simulink model "sedemo_batch_production"  (Simulink 7.5)
settings: Solver=VariableStepDiscrete  StartTime=0.0  StopTime=1000  MaxStep=inf  RelTol=1e-3
PreLoadFcn:
  | assignin('base','AGenerationPeriod',10);
  | assignin('base','AServiceTimeWater',10);
  | assignin('base','AServiceTimeHeat',20);
  | assignin('base','AServiceTimeColor',3);
  | assignin('base','AServiceTimeParticle',5);
  | assignin('base','AServiceTimeStir',10);
  | assignin('base','AServiceTimeDrain',10);
  | assignin('base','BGenerationPeriod',15);
  | assignin('base','BServiceTimeWater',15);
  | assignin('base','BServiceTimeHeat',30);
  | assignin('base','BServiceTimeColor',6);
  | assignin('base','BServiceTimeParticle',10);
  | assignin('base','BServiceTimeStir',20);
  | assignin('base','BServiceTimeDrain',15);
  | assignin('base','NumberOfBatchReactors',10);
  | assignin('base','NumberOfWater',2);
  | assignin('base','NumberOfHeat',3);
  | assignin('base','NumberOfDrain',1);
undefined symbols (not defined in the file or in its folder): AGenerationPeriod, BGenerationPeriod, des_subsystemblock, des_subsysteminport, des_subsystemoutport, des_subsystemsupportblock, NumberOfBatchReactors
libraries: simeventssink1 x12, simeventsserver1 x6, simeventsqueue1 x5, simeventstranslate1 x4, simeventsgenerators1 x3, simeventsrouting1 x3, simeventsentitymanage1 x2, simeventsattributes2 x2, simulink x1, simeventsinfo x1
CloseFcn:
  | clear AGenerationPeriod AServiceTimeWater AServiceTimeHeat AServiceTimeColor AServiceTimeParticle AServiceTimeStir AServiceTimeDrain BGenerationPeriod BServiceTimeWater BServiceTimeHeat BServiceTimeColor BServiceTimeParticle BServiceTimeStir BServiceTimeDrain NumberOfBatchReactors NumberOfHeat NumberOfWater NumberOfDrain;
settings Model: Creator=The MathWorks Inc.
settings DataIOCC: SaveOutput=off  SaveTime=off
settings OptimizationCC: EfficientMapNaN2IntZero=off
settings DebuggingCC: AlgebraicLoopMsg=error  SolverPrmCheckMsg=none  StrictBusMsg=Warning
settings SimEventsCC: propDiagAttribOutput=1  propDiagFcnCallOutput=1  propDiagStatOutput=0

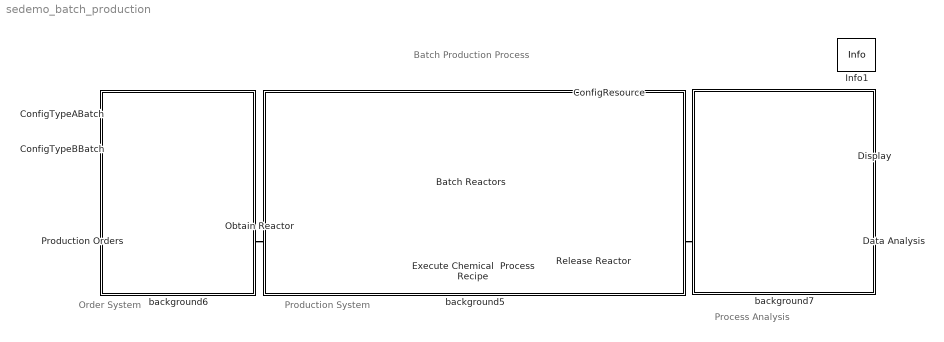
== system sedemo_batch_production ==
  note: Batch Production Process
  note: Production System
  note: Order System
  note: Process Analysis
  Batch Reactors : Subsystem
  ConfigResource : Subsystem  mask{NumBatchReactor=10, NumWater=2, NumHeat=3, NumDrain=1}
      mask prompts: NumBatchReactor "Number of batch reactors:"; NumWater "Capacity of water supply (number of reactors that can access simultaneously):"; NumHeat "Capacity of heat supply (number of reactors that can access simultaneously):"; NumDrain "Capacity of draining facility (number of reactors that can access simultaneously):"
      mask init:
      | assignin('base','NumberOfBatchReactors',NumBatchReactor);
      | assignin('base','NumberOfWater',NumWater);
      | assignin('base','NumberOfHeat',NumHeat);
      | assignin('base','NumberOfDrain',NumDrain);
      mask Display: disp('Double click here to configure\nresource capacity')
  ConfigTypeABatch : Subsystem  mask(Type A batch){AGenPeriod=10, ADelayWater=10, ADelayHeat=20, ADelayColor=3, ADelayParticle=5, ADelayStir=10, ADelayDrain=10}
      mask prompts: AGenPeriod "Order generation period of type A batch:"; ADelayWater "Time needed to add water:"; ADelayHeat "Time needed to heat up:"; ADelayColor "Time needed to add color:"; ADelayParticle "Time needed to add particles:"; ADelayStir "Time needed for agitation:"; ADelayDrain "Time needed to drain:"
      mask init:
      | assignin('base','AGenerationPeriod',AGenPeriod);
      | assignin('base','AServiceTimeWater',ADelayWater);
      | assignin('base','AServiceTimeHeat',ADelayHeat);
      | assignin('base','AServiceTimeColor',ADelayColor);
      | assignin('base','AServiceTimeParticle',ADelayParticle);
      | assignin('base','AServiceTimeStir',ADelayStir);
      | assignin('base','AServiceTimeDrain',ADelayDrain);
      mask Display: disp('Double click here to configure\ntype A batch')
  ConfigTypeBBatch : Subsystem  mask(Type B Batch){BGenPeriod=15, BDelayWater=15, BDelayHeat=30, BDelayColor=6, BDelayParticle=10, BDelayStir=20, BDelayDrain=15}
      mask prompts: BGenPeriod "Order generation period of type B batch:"; BDelayWater "Time needed to add water:"; BDelayHeat "Time needed to heat up:"; BDelayColor "Time needed to add color:"; BDelayParticle "Time needed to add particles:"; BDelayStir "Time needed for agitation:"; BDelayDrain "Time needed to drain:"
      mask init:
      | assignin('base','BGenerationPeriod',BGenPeriod);
      | assignin('base','BServiceTimeWater',BDelayWater);
      | assignin('base','BServiceTimeHeat',BDelayHeat);
      | assignin('base','BServiceTimeColor',BDelayColor);
      | assignin('base','BServiceTimeParticle',BDelayParticle);
      | assignin('base','BServiceTimeStir',BDelayStir);
      | assignin('base','BServiceTimeDrain',BDelayDrain);
      mask Display: disp('Double click here to configure\ntype B batch')
  Data Analysis : Subsystem
  Display : Display
  Execute Chemical  Process Recipe : Subsystem
      mask Display: image(imread('sedemo_batch_reactor.jpg'));
  Info1 : simeventsinfo/Info  SystemSampleTime=-1
  Obtain Reactor : simeventsentitymanage1/Entity Combiner  Priority=1  SystemSampleTime=-1  NumberInputPorts=2  RetainComponentEntities=on  AttributeAccessibility=on  TimerAccessibility=on  AttributeCopied=on  TimerCopied=on  StatNumberDeparted=Off  EvaluatedNumPorts=2
  Production Orders : Subsystem
  Release Reactor : simeventsentitymanage1/Entity Splitter  Priority=1  SystemSampleTime=-1  NumberOutputPorts=2  SplitEntityWhen=All entity output ports are not blocked  OutputPortPrecedence=OUT1 port  InitialSeed=56789  ActionUponPortMismatch=Continue  ActionUponBlocking=Discard entity  StatNumberArrived=Off  StatNumberDeparted=Off  EvaluatedNumPorts=2
  background5 : Subsystem
      mask Display: disp('')
  background6 : Subsystem
      mask Display: disp('')
  background7 : Subsystem
      mask Display:
      | text(18,170,'Reactor util:');
      | text(18,150,'Water util:');
      | text(18,130,'Heat util:');
      | text(18,110,'Drain util:');
  wires:
  Data Analysis/1(ResourceUtil) -> Display/1
  connections:
  Obtain Reactor/RConn1 -- Execute Chemical  Process Recipe/LConn1
  Execute Chemical  Process Recipe/RConn1 -- Release Reactor/LConn1
  Obtain Reactor/LConn1 -- Batch Reactors/RConn1
  Batch Reactors/LConn1 -- Release Reactor/RConn1
  Release Reactor/RConn2 -- Data Analysis/LConn1
  Production Orders/RConn1 -- Obtain Reactor/LConn2

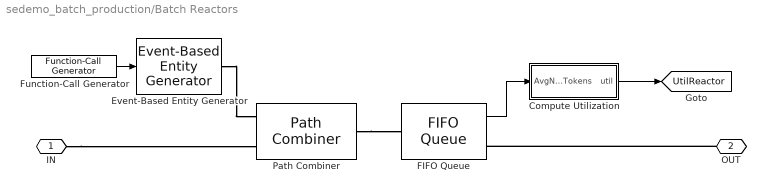
== system sedemo_batch_production/Batch Reactors ==
  Compute Utilization : Subsystem
  Event-Based Entity Generator : simeventsgenerators1/Entity Generators/Event-Based Entity Generator  Priority=1  DialogController=des_ddg_create  DialogControllerArgs=DataTag10  SystemSampleTime=-1  GenerateEntitiesUpon=Function call from port fcn  SignalEdgeType=Rising  SpecifyEventPriority=off  PriorityEntityGeneration=300  GenerateEntityAtSimulationStart=on  AllowBlocking=on  ResponseDuringBlockage=Discard generated entities  EntityType=Blank  StatNumberDeparted=Off  StatPendingEntity=Off  StatAverageIntergenerationTime=Off
  FIFO Queue : simeventsqueue1/FIFO Queue  Priority=1  SystemSampleTime=-1  Capacity=Inf  EnableTOPort=off  StatNumberDeparted=Off  StatNumberInBlock=Off  StatPendingEntity=Off  StatAverageWait=Off  StatAverageQueueLength=On  StatNumberTimedout=Off
  Function-Call Generator : simulink/Ports & Subsystems/Function-Call Generator  sample_time=1e8  numberOfIterations=NumberOfBatchReactors
  Path Combiner : simeventsrouting1/Path Combiner  Priority=1  SystemSampleTime=-1  NumberInputPorts=2  InputPortPrecedence=IN1 port  InitialSeed=45675  SpecifyEventPriority=off  PriorityPathCombinerPortPrecedenceSelection=4100  StatNumberDeparted=Off  StatLastArrivalPort=Off  EvaluatedNumPorts=2
  IN : PMIOPort  Port=1  Side=Left
  OUT : PMIOPort  Port=2  Side=Right
  tag scope: UtilReactor=global
  wires:
  Function-Call Generator/1 -> Event-Based Entity Generator/1
  FIFO Queue/1 -> Compute Utilization/1(AvgNumTokens)
  Compute Utilization/1(util) -> [UtilReactor]
  connections:
  OUT/RConn1 -- FIFO Queue/RConn1
  Path Combiner/RConn1 -- FIFO Queue/LConn1
  Event-Based Entity Generator/RConn1 -- Path Combiner/LConn1
  IN/RConn1 -- Path Combiner/LConn2

== system sedemo_batch_production/ConfigResource ==

== system sedemo_batch_production/ConfigTypeABatch ==

== system sedemo_batch_production/ConfigTypeBBatch ==

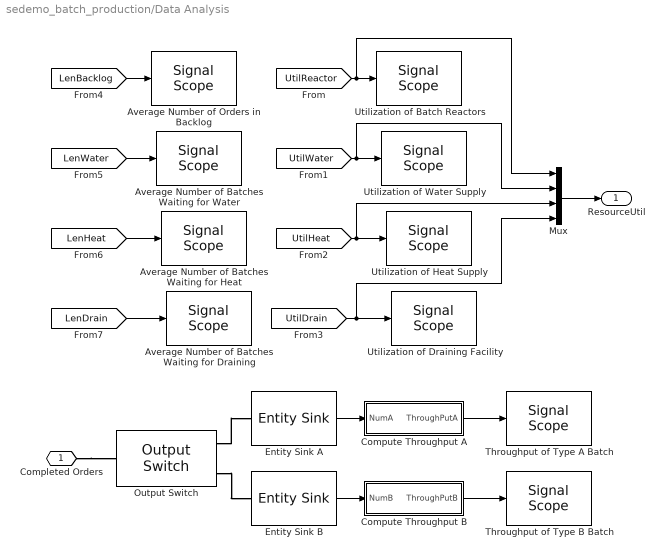
== system sedemo_batch_production/Data Analysis ==
  Average Number of Batches Waiting for Draining : simeventssink1/Signal Scope  Priority=1  SystemSampleTime=-1  PlotType=Stair  InputType=Signal  NumInputs=1  AttributeNameY=Count  XInputOptionSignal=Event time  XInputOptionEntity=Event time  AttributeNameX=Count  EnableEntityOutport=on  XMin=0  XMax=1000  XLimitExceededOption=Stretch axis limits  YLimitExceededOption=Stretch axis limits  AxisGrid=on  AxisLegend=off  LineDisables=""  LineColors=b  LineStyles=-  LineMarkers=None  OpenScopeAtSimStart=on  Title=Avg Num of Batches Waiting for Draining  YLabel=Count  XLabel=Time  FigurePosition=[50 32 259 136]  AxisZoom=off  DataStoreOption=Limited  DataPointsLimit=10000  StatNumberArrived=Off  ShowCountPlotted=off  ShowToolbar=off
      settings: YMin=0  YMax=2
  Average Number of Batches Waiting for Heat : simeventssink1/Signal Scope  Priority=1  SystemSampleTime=-1  PlotType=Stair  InputType=Signal  NumInputs=1  AttributeNameY=Count  XInputOptionSignal=Event time  XInputOptionEntity=Event time  AttributeNameX=Count  EnableEntityOutport=on  XMin=0  XMax=1000  XLimitExceededOption=Stretch axis limits  YLimitExceededOption=Stretch axis limits  AxisGrid=on  AxisLegend=off  LineDisables=""  LineColors="0  1  0"  LineStyles=-  LineMarkers=None  OpenScopeAtSimStart=on  Title=Avg Num of Batches waiting for Heat  YLabel=Count  XLabel=Time  FigurePosition=[50 216 259 136]  AxisZoom=off  DataStoreOption=Limited  DataPointsLimit=10000  StatNumberArrived=Off  ShowCountPlotted=off  ShowToolbar=off
      settings: YMin=0  YMax=2
  Average Number of Batches Waiting for Water : simeventssink1/Signal Scope  Priority=1  SystemSampleTime=-1  PlotType=Stair  InputType=Signal  NumInputs=1  AttributeNameY=Count  XInputOptionSignal=Event time  XInputOptionEntity=Event time  AttributeNameX=Count  EnableEntityOutport=on  XMin=0  XMax=1000  XLimitExceededOption=Stretch axis limits  YLimitExceededOption=Stretch axis limits  AxisGrid=on  AxisLegend=off  LineDisables=""  LineColors="1  0  1"  LineStyles=-  LineMarkers=None  OpenScopeAtSimStart=on  Title=Avg Num of Batches Waiting for Water  YLabel=Count  XLabel=Time  FigurePosition=[52 399 258 136]  AxisZoom=off  DataStoreOption=Limited  DataPointsLimit=10000  StatNumberArrived=Off  ShowCountPlotted=off  ShowToolbar=off
      settings: YMin=0  YMax=2
  Average Number of Orders in Backlog : simeventssink1/Signal Scope  Priority=1  SystemSampleTime=-1  PlotType=Stair  InputType=Signal  NumInputs=1  AttributeNameY=Count  XInputOptionSignal=Event time  XInputOptionEntity=Event time  AttributeNameX=Count  EnableEntityOutport=on  XMin=0  XMax=1000  XLimitExceededOption=Stretch axis limits  YLimitExceededOption=Stretch axis limits  AxisGrid=on  AxisLegend=off  LineDisables=""  LineColors="1  0  0"  LineStyles=-  LineMarkers=None  OpenScopeAtSimStart=on  Title=Average Volume of Order Backlog  YLabel=Count  XLabel=Time  FigurePosition=[51 583 259 136]  AxisZoom=off  DataStoreOption=Limited  DataPointsLimit=10000  StatNumberArrived=Off  ShowCountPlotted=off  ShowToolbar=off
      settings: YMin=0  YMax=2
  Compute Throughput A : Subsystem  LoadFcn=des_subsystemblock(gcb, 'load');  InitFcn=des_subsystemblock(gcb, 'init');  StartFcn=des_subsystemblock(gcb, 'start');  StopFcn=des_subsystemblock(gcb, 'stop');
      settings: CopyFcn=des_subsystemblock(gcb, 'copy');  DeleteFcn=des_subsystemblock(gcb, 'delete');  UndoDeleteFcn=des_subsystemblock(gcb, 'undodelete');  ModelCloseFcn=des_subsystemblock(gcb, 'modelclose');  PreSaveFcn=des_subsystemblock(gcb, 'presave');  NameChangeFcn=des_subsystemblock(gcb, 'namechange');  OpenFcn=des_subsystemblock(gcb, 'open');  ParentCloseFcn=des_subsystemblock(gcb, 'parentclose');  ErrorFcn=des_subsystemerror
      mask Type: Discrete Event Subsystem
      mask Help: helpview(simeventsbhelp);
  Compute Throughput B : Subsystem  LoadFcn=des_subsystemblock(gcb, 'load');  InitFcn=des_subsystemblock(gcb, 'init');  StartFcn=des_subsystemblock(gcb, 'start');  StopFcn=des_subsystemblock(gcb, 'stop');
      settings: CopyFcn=des_subsystemblock(gcb, 'copy');  DeleteFcn=des_subsystemblock(gcb, 'delete');  UndoDeleteFcn=des_subsystemblock(gcb, 'undodelete');  ModelCloseFcn=des_subsystemblock(gcb, 'modelclose');  PreSaveFcn=des_subsystemblock(gcb, 'presave');  NameChangeFcn=des_subsystemblock(gcb, 'namechange');  OpenFcn=des_subsystemblock(gcb, 'open');  ParentCloseFcn=des_subsystemblock(gcb, 'parentclose');  ErrorFcn=des_subsystemerror
      mask Type: Discrete Event Subsystem
      mask Help: helpview(simeventsbhelp);
  Entity Sink A : simeventssink1/Entity Sink  Priority=1  SystemSampleTime=-1  AvailableForArrivals=on  StatNumberArrived=On
  Entity Sink B : simeventssink1/Entity Sink  Priority=1  SystemSampleTime=-1  AvailableForArrivals=on  StatNumberArrived=On
  Mux : Mux
  Output Switch : simeventsrouting1/Output Switch  Priority=1  SystemSampleTime=-1  NumberOutputPorts=2  SwitchingCriterion=From attribute  InitialSeed=34567  AttributeName=TypeOfBatch  InitialConditionsOpt=off  InitialConditions=1  EntityBufferOpt=off  SpecifyEventPriority=off  PriorityOutputSwitchSelectPort=4100  TimeoutPortOpt=off  StatNumberDeparted=Off  StatNumberTimedOut=Off  StatPendingEntity=Off  StatLastDeparturePort=Off  EvaluatedNumPorts=2
  Throughput of Type A Batch : simeventssink1/Signal Scope  Priority=1  SystemSampleTime=-1  PlotType=Stair  InputType=Signal  NumInputs=1  AttributeNameY=Count  XInputOptionSignal=Event time  XInputOptionEntity=Event time  AttributeNameX=Count  EnableEntityOutport=on  XMin=0  XMax=1000  XLimitExceededOption=Stretch axis limits  YLimitExceededOption=Stretch axis limits  AxisGrid=on  AxisLegend=off  LineDisables=""  LineColors=b  LineStyles=-  LineMarkers=None  OpenScopeAtSimStart=on  Title=Throughput of Type A Batch  YLabel=Throughput (batch/sec)  XLabel=Time  FigurePosition=[606 404 285 146]  AxisZoom=off  DataStoreOption=Limited  DataPointsLimit=10000  StatNumberArrived=Off  ShowCountPlotted=off  ShowToolbar=off
      settings: YMin=0  YMax=0.1
  Throughput of Type B Batch : simeventssink1/Signal Scope  Priority=1  SystemSampleTime=-1  PlotType=Stair  InputType=Signal  NumInputs=1  AttributeNameY=Count  XInputOptionSignal=Event time  XInputOptionEntity=Event time  AttributeNameX=Count  EnableEntityOutport=on  XMin=0  XMax=1000  XLimitExceededOption=Stretch axis limits  YLimitExceededOption=Stretch axis limits  AxisGrid=on  AxisLegend=off  LineDisables=""  LineColors=b  LineStyles=-  LineMarkers=None  OpenScopeAtSimStart=on  Title=Throughput of Type B Batch  YLabel=Throughput (batch/sec)  XLabel=Time  FigurePosition=[606 211 285 146]  AxisZoom=off  DataStoreOption=Limited  DataPointsLimit=10000  StatNumberArrived=Off  ShowCountPlotted=off  ShowToolbar=off
      settings: YMin=0  YMax=0.1
  Utilization of Batch Reactors : simeventssink1/Signal Scope  Priority=1  SystemSampleTime=-1  PlotType=Stair  InputType=Signal  NumInputs=1  AttributeNameY=Count  XInputOptionSignal=Event time  XInputOptionEntity=Event time  AttributeNameX=Count  EnableEntityOutport=on  XMin=0  XMax=1000  XLimitExceededOption=Stretch axis limits  YLimitExceededOption=Stretch axis limits  AxisGrid=on  AxisLegend=off  LineDisables=""  LineColors="1  0  0"  LineStyles=-  LineMarkers=None  OpenScopeAtSimStart=on  Title=Utilization of Batch Reactors  YLabel=Utilization  XLabel=Time  FigurePosition=[318 584 264 135]  AxisZoom=off  DataStoreOption=Limited  DataPointsLimit=10000  StatNumberArrived=Off  ShowCountPlotted=off  ShowToolbar=off
      settings: YMin=0  YMax=1.2
  Utilization of Draining Facility : simeventssink1/Signal Scope  Priority=1  SystemSampleTime=-1  PlotType=Stair  InputType=Signal  NumInputs=1  AttributeNameY=Count  XInputOptionSignal=Event time  XInputOptionEntity=Event time  AttributeNameX=Count  EnableEntityOutport=on  XMin=0  XMax=1000  XLimitExceededOption=Stretch axis limits  YLimitExceededOption=Stretch axis limits  AxisGrid=on  AxisLegend=off  LineDisables=""  LineColors=b  LineStyles=-  LineMarkers=None  OpenScopeAtSimStart=on  Title=Utilization of Draining Facility  YLabel=Utilization  XLabel=Time  FigurePosition=[317 33 265 135]  AxisZoom=off  DataStoreOption=Limited  DataPointsLimit=10000  StatNumberArrived=Off  ShowCountPlotted=off  ShowToolbar=off
      settings: YMin=0  YMax=1.2
  Utilization of Heat Supply : simeventssink1/Signal Scope  Priority=1  SystemSampleTime=-1  PlotType=Stair  InputType=Signal  NumInputs=1  AttributeNameY=Count  XInputOptionSignal=Event time  XInputOptionEntity=Event time  AttributeNameX=Count  EnableEntityOutport=on  XMin=0  XMax=1000  XLimitExceededOption=Stretch axis limits  YLimitExceededOption=Stretch axis limits  AxisGrid=on  AxisLegend=off  LineDisables=""  LineColors="0  1  0"  LineStyles=-  LineMarkers=None  OpenScopeAtSimStart=on  Title=Utilization of Heat  YLabel=Utilization  XLabel=Time  FigurePosition=[317 216 265 137]  AxisZoom=off  DataStoreOption=Limited  DataPointsLimit=10000  StatNumberArrived=Off  ShowCountPlotted=off  ShowToolbar=off
      settings: YMin=0  YMax=1.2
  Utilization of Water Supply : simeventssink1/Signal Scope  Priority=1  SystemSampleTime=-1  PlotType=Stair  InputType=Signal  NumInputs=1  AttributeNameY=Count  XInputOptionSignal=Event time  XInputOptionEntity=Event time  AttributeNameX=Count  EnableEntityOutport=on  XMin=0  XMax=1000  XLimitExceededOption=Stretch axis limits  YLimitExceededOption=Stretch axis limits  AxisGrid=on  AxisLegend=off  LineDisables=""  LineColors="1  0  1"  LineStyles=-  LineMarkers=None  OpenScopeAtSimStart=on  Title=Utilization of Water  YLabel=Utilization  XLabel=Time  FigurePosition=[318 401 264 135]  AxisZoom=off  DataStoreOption=Limited  DataPointsLimit=10000  StatNumberArrived=Off  ShowCountPlotted=off  ShowToolbar=off
      settings: YMin=0  YMax=1.2
  Completed Orders : PMIOPort  Port=1  Side=Left
  ResourceUtil : Outport  OutDataType=sfix(16)  OutScaling=2^0
  wires:
  [UtilReactor] -> Utilization of Batch Reactors/1, Mux/1
  [UtilWater] -> Utilization of Water Supply/1, Mux/2
  [UtilDrain] -> Utilization of Draining Facility/1, Mux/4
  [UtilHeat] -> Utilization of Heat Supply/1, Mux/3
  [LenBacklog] -> Average Number of Orders in Backlog/1
  [LenWater] -> Average Number of Batches Waiting for Water/1
  [LenDrain] -> Average Number of Batches Waiting for Draining/1
  [LenHeat] -> Average Number of Batches Waiting for Heat/1
  Entity Sink A/1 -> Compute Throughput A/1(NumA)
  Entity Sink B/1 -> Compute Throughput B/1(NumB)
  Compute Throughput A/1(ThroughPutA) -> Throughput of Type A Batch/1
  Compute Throughput B/1(ThroughPutB) -> Throughput of Type B Batch/1
  Mux/1 -> ResourceUtil/1
  connections:
  Completed Orders/RConn1 -- Output Switch/LConn1
  Output Switch/RConn1 -- Entity Sink A/LConn1
  Output Switch/RConn2 -- Entity Sink B/LConn1

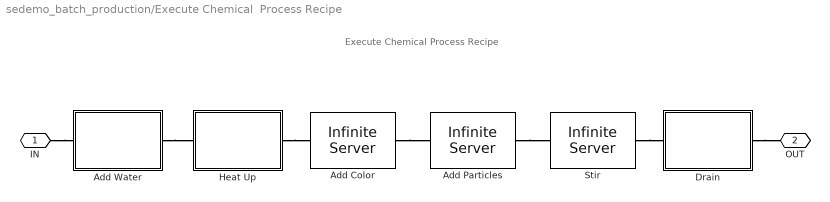
== system sedemo_batch_production/Execute Chemical  Process Recipe ==
  note: Execute Chemical Process Recipe
  Add Color : simeventsserver1/Infinite Server  Priority=1  SystemSampleTime=-1  ServiceTimeFrom=Attribute  ServiceTime=1  AttributeName=ServiceTimeColor  PriorityServiceCompletion=500  EnableTOPort=off  StatNumberDeparted=Off  StatNumberInBlock=Off  StatPendingEntity=Off  StatNumberPending=Off  StatAverageWait=Off  StatNumberTimedout=Off
  Add Particles : simeventsserver1/Infinite Server  Priority=1  SystemSampleTime=-1  ServiceTimeFrom=Attribute  ServiceTime=1  AttributeName=ServiceTimeParticle  PriorityServiceCompletion=500  EnableTOPort=off  StatNumberDeparted=Off  StatNumberInBlock=Off  StatPendingEntity=Off  StatNumberPending=Off  StatAverageWait=Off  StatNumberTimedout=Off
  Add Water : Subsystem
  Drain : Subsystem
  Heat Up : Subsystem
  Stir : simeventsserver1/Infinite Server  Priority=1  SystemSampleTime=-1  ServiceTimeFrom=Attribute  ServiceTime=1  AttributeName=ServiceTimeStir  PriorityServiceCompletion=500  EnableTOPort=off  StatNumberDeparted=Off  StatNumberInBlock=Off  StatPendingEntity=Off  StatNumberPending=Off  StatAverageWait=Off  StatNumberTimedout=Off
  IN : PMIOPort  Port=1  Side=Left
  OUT : PMIOPort  Port=2  Side=Right
  connections:
  Add Color/RConn1 -- Add Particles/LConn1
  Add Particles/RConn1 -- Stir/LConn1
  IN/RConn1 -- Add Water/LConn1
  Add Water/RConn1 -- Heat Up/LConn1
  Heat Up/RConn1 -- Add Color/LConn1
  Stir/RConn1 -- Drain/LConn1
  Drain/RConn1 -- OUT/RConn1

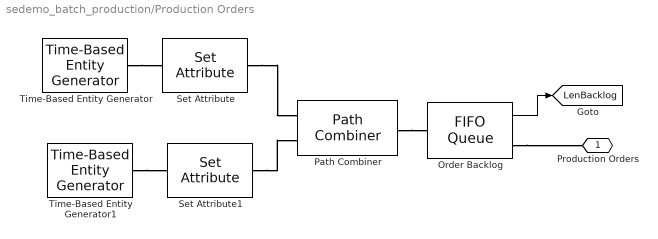
== system sedemo_batch_production/Production Orders ==
  Order Backlog : simeventsqueue1/FIFO Queue  Priority=1  SystemSampleTime=-1  Capacity=Inf  EnableTOPort=off  StatNumberDeparted=Off  StatNumberInBlock=Off  StatPendingEntity=Off  StatAverageWait=Off  StatAverageQueueLength=On  StatNumberTimedout=Off
  Path Combiner : simeventsrouting1/Path Combiner  Priority=1  SystemSampleTime=-1  NumberInputPorts=2  InputPortPrecedence=IN1 port  InitialSeed=45675  SpecifyEventPriority=off  PriorityPathCombinerPortPrecedenceSelection=4100  StatNumberDeparted=Off  StatLastArrivalPort=Off  EvaluatedNumPorts=2
  Set Attribute : simeventsattributes2/Set Attribute  Priority=1  DialogController=des_ddg_create  DialogControllerArgs=DataTag53  SystemSampleTime=-1  AttributeFrom=Dialog|Dialog|Dialog|Dialog|Dialog|Dialog|Dialog  AttributeName=ServiceTimeWater|ServiceTimeHeat|ServiceTimeColor|ServiceTimeParticle|ServiceTimeStir|ServiceTimeDrain|TypeOfBatch  AttributeTreatAsVector=1|1|1|1|1|1|1  AttributeValue=AServiceTimeWater|AServiceTimeHeat|AServiceTimeColor|AServiceTimeParticle|AServiceTimeStir|AServiceTimeDrain|1  AttributeCreate=on  StatNumberDeparted=Off  EvaluatedAttributeValue={AServiceTimeWater;AServiceTimeHeat;AServiceTimeColor;AServiceTimeParticle;AServiceTimeStir;AServiceTimeDrain;1}
  Set Attribute1 : simeventsattributes2/Set Attribute  Priority=1  DialogController=des_ddg_create  DialogControllerArgs=DataTag55  SystemSampleTime=-1  AttributeFrom=Dialog|Dialog|Dialog|Dialog|Dialog|Dialog|Dialog  AttributeName=ServiceTimeWater|ServiceTimeHeat|ServiceTimeColor|ServiceTimeParticle|ServiceTimeStir|ServiceTimeDrain|TypeOfBatch  AttributeTreatAsVector=1|1|1|1|1|1|1  AttributeValue=BServiceTimeWater|BServiceTimeHeat|BServiceTimeColor|BServiceTimeParticle|BServiceTimeStir|BServiceTimeDrain|2  AttributeCreate=on  StatNumberDeparted=Off  EvaluatedAttributeValue={BServiceTimeWater;BServiceTimeHeat;BServiceTimeColor;BServiceTimeParticle;BServiceTimeStir;BServiceTimeDrain;2}
  Time-Based Entity Generator : simeventsgenerators1/Entity Generators/Time-Based Entity Generator  Priority=1  DialogController=des_ddg_create  DialogControllerArgs=DataTag57  SystemSampleTime=-1  GenerateEntitiesUpon=Intergeneration time from dialog  Distribution=Constant  Minimum=0  Maximum=1  Mean=1  InitialSeed=12345  Period=AGenerationPeriod  PriorityEntityGeneration=300  GenerateEntityAtSimulationStart=off  ResponseWhenBlocked=Pause generation  ResponseWhenUnblocked=Immediate restart  EntityType=Blank  StatNumberDeparted=Off  StatPendingEntity=Off  StatAverageIntergenerationTime=Off
  Time-Based Entity Generator1 : simeventsgenerators1/Entity Generators/Time-Based Entity Generator  Priority=1  DialogController=des_ddg_create  DialogControllerArgs=DataTag59  SystemSampleTime=-1  GenerateEntitiesUpon=Intergeneration time from dialog  Distribution=Constant  Minimum=0  Maximum=1  Mean=1  InitialSeed=12345  Period=BGenerationPeriod  PriorityEntityGeneration=300  GenerateEntityAtSimulationStart=off  ResponseWhenBlocked=Pause generation  ResponseWhenUnblocked=Immediate restart  EntityType=Blank  StatNumberDeparted=Off  StatPendingEntity=Off  StatAverageIntergenerationTime=Off
  Production Orders : PMIOPort  Port=1  Side=Right
  tag scope: LenBacklog=global
  wires:
  Order Backlog/1 -> [LenBacklog]
  connections:
  Set Attribute/RConn1 -- Path Combiner/LConn1
  Set Attribute1/RConn1 -- Path Combiner/LConn2
  Time-Based Entity Generator/RConn1 -- Set Attribute/LConn1
  Time-Based Entity Generator1/RConn1 -- Set Attribute1/LConn1
  Path Combiner/RConn1 -- Order Backlog/LConn1
  Order Backlog/RConn1 -- Production Orders/RConn1

== system sedemo_batch_production/background5 ==

== system sedemo_batch_production/background6 ==

== system sedemo_batch_production/background7 ==

== system sedemo_batch_production/Batch Reactors/Compute Utilization ==
  AvgNumTokens : Inport
  Constant : Constant  Value=NumberOfBatchReactors  OutDataType=sfix(16)  OutScaling=2^0
  Discrete Event Subsystem : Subsystem  LoadFcn=des_subsystemblock(gcb, 'load');  InitFcn=des_subsystemblock(gcb, 'init');  StartFcn=des_subsystemblock(gcb, 'start');  StopFcn=des_subsystemblock(gcb, 'stop');
      settings: CopyFcn=des_subsystemblock(gcb, 'copy');  DeleteFcn=des_subsystemblock(gcb, 'delete');  UndoDeleteFcn=des_subsystemblock(gcb, 'undodelete');  ModelCloseFcn=des_subsystemblock(gcb, 'modelclose');  PreSaveFcn=des_subsystemblock(gcb, 'presave');  NameChangeFcn=des_subsystemblock(gcb, 'namechange');  OpenFcn=des_subsystemblock(gcb, 'open');  ParentCloseFcn=des_subsystemblock(gcb, 'parentclose');  ErrorFcn=des_subsystemerror
      mask Type: Discrete Event Subsystem
      mask Help: helpview(simeventsbhelp);
  util : Outport
  wires:
  Constant/1 -> Discrete Event Subsystem/1(Capacity)
  Discrete Event Subsystem/1(util) -> util/1
  AvgNumTokens/1 -> Discrete Event Subsystem/2(AvgNumTokens)

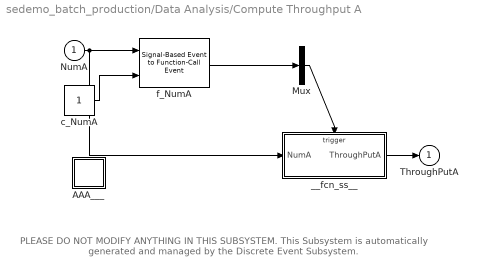
== system sedemo_batch_production/Data Analysis/Compute Throughput A ==
  note: PLEASE DO NOT MODIFY ANYTHING IN THIS SUBSYSTEM.
      | This Subsystem is automatically generated and
      | managed by the Discrete Event Subsystem.
  NumA : Inport  DataType=double  OutDataType=sfix(16)  OutScaling=2^0  OutDataTypeStr=double
  AAA___ : Subsystem  LoadFcn=des_subsystemsupportblock(gcb, 'load');  InitFcn=des_subsystemsupportblock(gcb, 'init');  StartFcn=des_subsystemsupportblock(gcb, 'start');  StopFcn=des_subsystemsupportblock(gcb, 'stop');
      settings: CopyFcn=des_subsystemsupportblock(gcb, 'copy');  DeleteFcn=des_subsystemsupportblock(gcb, 'delete');  UndoDeleteFcn=des_subsystemsupportblock(gcb, 'undodelete');  ModelCloseFcn=des_subsystemsupportblock(gcb, 'modelclose');  PreSaveFcn=des_subsystemsupportblock(gcb, 'presave');  NameChangeFcn=des_subsystemsupportblock(gcb, 'namechange');  OpenFcn=des_subsystemsupportblock(gcb, 'open');  ParentCloseFcn=des_subsystemsupportblock(gcb, 'parentclose');
  Mux : Mux  Inputs=1
  __fcn_ss__ : Subsystem  TreatAsAtomicUnit=on
      settings: PropExecContextOutsideSubsystem=on
  c_NumA : Constant  OutDataType=sfix(16)  OutScaling=2^0
  f_NumA : simeventstranslate1/Signal-Based Event to Function-Call Event  Priority=1  SystemSampleTime=-1  GenerateFunctionCallUpon=Sample time hit from port ts  SignalEdgeOption=Rising  EnableE1Port=on  EnableF2Port=off  EnableE2Port=off  SpecifyEventPriority=off  PriorityFunctionCall=20  FunctionCallDelayFrom=Dialog  DelayFunctionCall=0  StatNumberF1Calls=Off  StatNumberF2Calls=Off  MaskBlockType=DESS_EVENT_PORT
  ThroughPutA : Outport  OutDataType=sfix(16)  OutScaling=2^0
  wires:
  __fcn_ss__/1(ThroughPutA) -> ThroughPutA/1
  f_NumA/1 -> Mux/1
  c_NumA/1 -> f_NumA/2
  Mux/1 -> __fcn_ss__/Trigger
  NumA/1 -> f_NumA/1, __fcn_ss__/1(NumA)

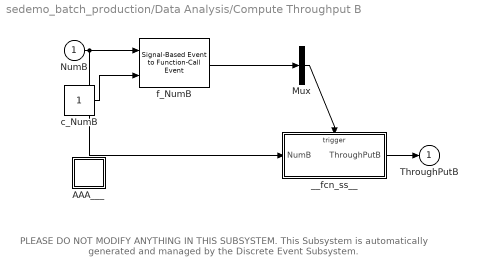
== system sedemo_batch_production/Data Analysis/Compute Throughput B ==
  note: PLEASE DO NOT MODIFY ANYTHING IN THIS SUBSYSTEM.
      | This Subsystem is automatically generated and
      | managed by the Discrete Event Subsystem.
  NumB : Inport  DataType=double  OutDataType=sfix(16)  OutScaling=2^0  OutDataTypeStr=double
  AAA___ : Subsystem  LoadFcn=des_subsystemsupportblock(gcb, 'load');  InitFcn=des_subsystemsupportblock(gcb, 'init');  StartFcn=des_subsystemsupportblock(gcb, 'start');  StopFcn=des_subsystemsupportblock(gcb, 'stop');
      settings: CopyFcn=des_subsystemsupportblock(gcb, 'copy');  DeleteFcn=des_subsystemsupportblock(gcb, 'delete');  UndoDeleteFcn=des_subsystemsupportblock(gcb, 'undodelete');  ModelCloseFcn=des_subsystemsupportblock(gcb, 'modelclose');  PreSaveFcn=des_subsystemsupportblock(gcb, 'presave');  NameChangeFcn=des_subsystemsupportblock(gcb, 'namechange');  OpenFcn=des_subsystemsupportblock(gcb, 'open');  ParentCloseFcn=des_subsystemsupportblock(gcb, 'parentclose');
  Mux : Mux  Inputs=1
  __fcn_ss__ : Subsystem  TreatAsAtomicUnit=on
      settings: PropExecContextOutsideSubsystem=on
  c_NumB : Constant  OutDataType=sfix(16)  OutScaling=2^0
  f_NumB : simeventstranslate1/Signal-Based Event to Function-Call Event  Priority=1  SystemSampleTime=-1  GenerateFunctionCallUpon=Sample time hit from port ts  SignalEdgeOption=Rising  EnableE1Port=on  EnableF2Port=off  EnableE2Port=off  SpecifyEventPriority=off  PriorityFunctionCall=20  FunctionCallDelayFrom=Dialog  DelayFunctionCall=0  StatNumberF1Calls=Off  StatNumberF2Calls=Off  MaskBlockType=DESS_EVENT_PORT
  ThroughPutB : Outport  OutDataType=sfix(16)  OutScaling=2^0
  wires:
  Mux/1 -> __fcn_ss__/Trigger
  c_NumB/1 -> f_NumB/2
  f_NumB/1 -> Mux/1
  __fcn_ss__/1(ThroughPutB) -> ThroughPutB/1
  NumB/1 -> f_NumB/1, __fcn_ss__/1(NumB)

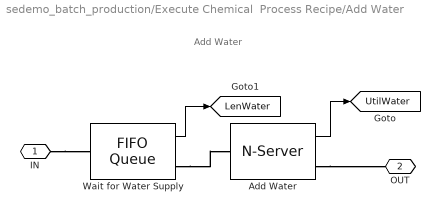
== system sedemo_batch_production/Execute Chemical  Process Recipe/Add Water ==
  note: Add Water
  Add Water : simeventsserver1/N-Server  Priority=1  SystemSampleTime=-1  NumberOfServers=NumberOfWater  ServiceTimeFrom=Attribute  ServiceTime=1  AttributeName=ServiceTimeWater  PriorityServiceCompletion=500  EnableTOPort=off  StatNumberDeparted=Off  StatNumberInBlock=Off  StatPendingEntity=Off  StatNumberPending=Off  StatAverageWait=Off  StatUtilization=On  StatNumberTimedout=Off
  Wait for Water Supply : simeventsqueue1/FIFO Queue  Priority=1  SystemSampleTime=-1  Capacity=Inf  EnableTOPort=off  StatNumberDeparted=Off  StatNumberInBlock=Off  StatPendingEntity=Off  StatAverageWait=Off  StatAverageQueueLength=On  StatNumberTimedout=Off
  IN : PMIOPort  Port=1  Side=Left
  OUT : PMIOPort  Port=2  Side=Right
  tag scope: LenWater=global, UtilWater=global
  wires:
  Add Water/1 -> [UtilWater]
  Wait for Water Supply/1 -> [LenWater]
  connections:
  Add Water/RConn1 -- OUT/RConn1
  IN/RConn1 -- Wait for Water Supply/LConn1
  Wait for Water Supply/RConn1 -- Add Water/LConn1

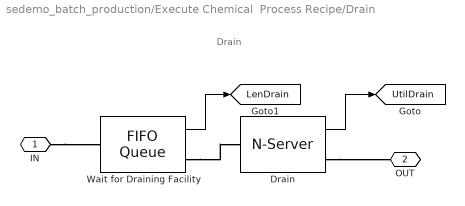
== system sedemo_batch_production/Execute Chemical  Process Recipe/Drain ==
  note: Drain
  Drain : simeventsserver1/N-Server  Priority=1  SystemSampleTime=-1  NumberOfServers=NumberOfDrain  ServiceTimeFrom=Attribute  ServiceTime=1  AttributeName=ServiceTimeDrain  PriorityServiceCompletion=500  EnableTOPort=off  StatNumberDeparted=Off  StatNumberInBlock=Off  StatPendingEntity=Off  StatNumberPending=Off  StatAverageWait=Off  StatUtilization=On  StatNumberTimedout=Off
  Wait for Draining Facility : simeventsqueue1/FIFO Queue  Priority=1  SystemSampleTime=-1  Capacity=Inf  EnableTOPort=off  StatNumberDeparted=Off  StatNumberInBlock=Off  StatPendingEntity=Off  StatAverageWait=Off  StatAverageQueueLength=On  StatNumberTimedout=Off
  IN : PMIOPort  Port=1  Side=Left
  OUT : PMIOPort  Port=2  Side=Right
  tag scope: LenDrain=global, UtilDrain=global
  wires:
  Drain/1 -> [UtilDrain]
  Wait for Draining Facility/1 -> [LenDrain]
  connections:
  IN/RConn1 -- Wait for Draining Facility/LConn1
  Wait for Draining Facility/RConn1 -- Drain/LConn1
  Drain/RConn1 -- OUT/RConn1

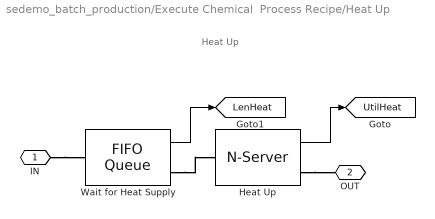
== system sedemo_batch_production/Execute Chemical  Process Recipe/Heat Up ==
  note: Heat Up
  Heat Up : simeventsserver1/N-Server  Priority=1  SystemSampleTime=-1  NumberOfServers=NumberOfHeat  ServiceTimeFrom=Attribute  ServiceTime=1  AttributeName=ServiceTimeHeat  PriorityServiceCompletion=500  EnableTOPort=off  StatNumberDeparted=Off  StatNumberInBlock=Off  StatPendingEntity=Off  StatNumberPending=Off  StatAverageWait=Off  StatUtilization=On  StatNumberTimedout=Off
  Wait for Heat Supply : simeventsqueue1/FIFO Queue  Priority=1  SystemSampleTime=-1  Capacity=Inf  EnableTOPort=off  StatNumberDeparted=Off  StatNumberInBlock=Off  StatPendingEntity=Off  StatAverageWait=Off  StatAverageQueueLength=On  StatNumberTimedout=Off
  IN : PMIOPort  Port=1  Side=Left
  OUT : PMIOPort  Port=2  Side=Right
  tag scope: LenHeat=global, UtilHeat=global
  wires:
  Heat Up/1 -> [UtilHeat]
  Wait for Heat Supply/1 -> [LenHeat]
  connections:
  Heat Up/RConn1 -- OUT/RConn1
  Wait for Heat Supply/RConn1 -- Heat Up/LConn1
  IN/RConn1 -- Wait for Heat Supply/LConn1

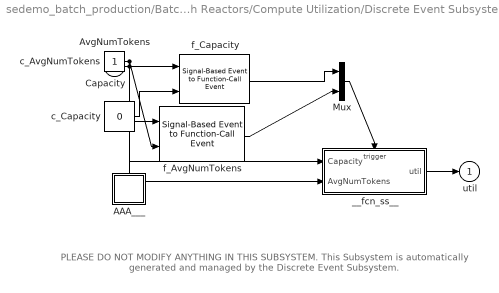
== system sedemo_batch_production/Batch Reactors/Compute Utilization/Discrete Event Subsystem ==
  note: PLEASE DO NOT MODIFY ANYTHING IN THIS SUBSYSTEM.
      | This Subsystem is automatically generated and
      | managed by the Discrete Event Subsystem.
  Capacity : Inport  DataType=double  OutDataType=sfix(16)  OutScaling=2^0  OutDataTypeStr=double
  AvgNumTokens : Inport  Port=2  DataType=double  OutDataTypeStr=double
  AAA___ : Subsystem  LoadFcn=des_subsystemsupportblock(gcb, 'load');  InitFcn=des_subsystemsupportblock(gcb, 'init');  StartFcn=des_subsystemsupportblock(gcb, 'start');  StopFcn=des_subsystemsupportblock(gcb, 'stop');
      settings: CopyFcn=des_subsystemsupportblock(gcb, 'copy');  DeleteFcn=des_subsystemsupportblock(gcb, 'delete');  UndoDeleteFcn=des_subsystemsupportblock(gcb, 'undodelete');  ModelCloseFcn=des_subsystemsupportblock(gcb, 'modelclose');  PreSaveFcn=des_subsystemsupportblock(gcb, 'presave');  NameChangeFcn=des_subsystemsupportblock(gcb, 'namechange');  OpenFcn=des_subsystemsupportblock(gcb, 'open');  ParentCloseFcn=des_subsystemsupportblock(gcb, 'parentclose');
  Mux : Mux  Inputs=2
  __fcn_ss__ : Subsystem  TreatAsAtomicUnit=on
      settings: PropExecContextOutsideSubsystem=on
  c_AvgNumTokens : Constant
  c_Capacity : Constant  Value=0  OutDataType=sfix(16)  OutScaling=2^0
  f_AvgNumTokens : simeventstranslate1/Signal-Based Event to Function-Call Event  Priority=1  SystemSampleTime=-1  GenerateFunctionCallUpon=Sample time hit from port ts  SignalEdgeOption=Rising  EnableE1Port=on  EnableF2Port=off  EnableE2Port=off  SpecifyEventPriority=off  PriorityFunctionCall=20  FunctionCallDelayFrom=Dialog  DelayFunctionCall=0  StatNumberF1Calls=Off  StatNumberF2Calls=Off  MaskBlockType=DESS_EVENT_PORT
  f_Capacity : simeventstranslate1/Signal-Based Event to Function-Call Event  Priority=1  SystemSampleTime=-1  GenerateFunctionCallUpon=Sample time hit from port ts  SignalEdgeOption=Rising  EnableE1Port=on  EnableF2Port=off  EnableE2Port=off  SpecifyEventPriority=off  PriorityFunctionCall=20  FunctionCallDelayFrom=Dialog  DelayFunctionCall=0  StatNumberF1Calls=Off  StatNumberF2Calls=Off  MaskBlockType=DESS_DATA_PORT
  util : Outport  OutDataType=sfix(16)  OutScaling=2^0
  wires:
  Capacity/1 -> __fcn_ss__/1(Capacity), f_Capacity/1
  __fcn_ss__/1(util) -> util/1
  f_Capacity/1 -> Mux/1
  c_Capacity/1 -> f_Capacity/2
  Mux/1 -> __fcn_ss__/Trigger
  f_AvgNumTokens/1 -> Mux/2
  c_AvgNumTokens/1 -> f_AvgNumTokens/2
  AvgNumTokens/1 -> f_AvgNumTokens/1, __fcn_ss__/2(AvgNumTokens)

== system sedemo_batch_production/Data Analysis/Compute Throughput A/AAA___ ==

== system sedemo_batch_production/Data Analysis/Compute Throughput A/__fcn_ss__ ==
  NumA : Inport  LoadFcn=des_subsysteminport(gcb, 'load');  InitFcn=des_subsysteminport(gcb, 'init');  StartFcn=des_subsysteminport(gcb, 'start');  StopFcn=des_subsysteminport(gcb, 'stop');  OutDataType=sfix(16)  OutScaling=2^0  mask(Discrete Event Inport){PermitSubsystemEvents=on, TypeOfEvent=Sample time hit, SignalEdgeOption=Rising, SpecifyEventPriority=off, PrioritySubsystemEvent=20}
      mask prompts: PermitSubsystemEvents "Execute subsystem upon signal-based events"; TypeOfEvent "Type of signal-based event:"; SignalEdgeOption "Type of change in signal value:"; SpecifyEventPriority "Resolve simultaneous signal updates according to event priority"; PrioritySubsystemEvent "Event priority:"
      mask help: Input port for a Discrete Event Subsystem block. This block can conditionally execute the subsystem upon signal-based events that meet specified criteria.
      mask init:
      | des_subsystemmask(gcb, 'init','apply')
      settings: CopyFcn=des_subsysteminport(gcb, 'copy');  DeleteFcn=des_subsysteminport(gcb, 'delete');  UndoDeleteFcn=des_subsysteminport(gcb, 'undodelete');  ModelCloseFcn=des_subsysteminport(gcb, 'modelclose');  PreSaveFcn=des_subsysteminport(gcb, 'presave');  NameChangeFcn=des_subsysteminport(gcb, 'namechange');  ParentCloseFcn=des_subsysteminport(gcb, 'parentclose');
      mask Help: helpview(simeventsbhelp);
      mask StyleString: checkbox,popup(Change in signal|Trigger|Sample time hit),popup(Rising|Falling|Either),checkbox,edit
      mask CallbackString: des_subsystemmask(gcb, 'cbPermitSubsystemEvents', 'noapply');|des_subsystemmask(gcb,'cbTypeOfEvent','noapply');||des_subsystemmask(gcb, 'cbSpecifyEventPriority', 'noapply');|
  Subsystem Configuration : TriggerPort  TriggerType=function-call
      settings: CopyFcn=des_subsystemconfigblock(gcb, 'copy');  DeleteFcn=des_subsystemconfigblock(gcb, 'delete');  UndoDeleteFcn=des_subsystemconfigblock(gcb, 'undodelete');
      mask Type: Subsystem Configuration
      mask Description: Configuration for a Discrete Event Subsystem block. Every discrete event subsystem window must contain exactly one copy of this configuration block. Do not delete this block.
      mask Help: helpview(simeventsbhelp);
      mask Display: disp('Do Not Delete');
  Digital Clock : DigitalClock  SampleTime=-1
  Divide : Product  Inputs=*/  OutDataType=sfix(16)  OutScaling=2^-10
  ThroughPutA : Outport  LoadFcn=des_subsystemoutport(gcb, 'load');  InitFcn=des_subsystemoutport(gcb, 'init');  StartFcn=des_subsystemoutport(gcb, 'start');  StopFcn=des_subsystemoutport(gcb, 'stop');  OutDataType=sfix(16)  OutScaling=2^0
      settings: CopyFcn=des_subsystemoutport(gcb, 'copy');  DeleteFcn=des_subsystemoutport(gcb, 'delete');  UndoDeleteFcn=des_subsystemoutport(gcb, 'undodelete');  ModelCloseFcn=des_subsystemoutport(gcb, 'modelclose');  PreSaveFcn=des_subsystemoutport(gcb, 'presave');  NameChangeFcn=des_subsystemoutport(gcb, 'namechange');  ParentCloseFcn=des_subsystemoutport(gcb, 'parentclose');
      mask Type: Discrete Event Outport
      mask Description: Provide an output port for a Discrete Event Subsystem block.
      mask Help: helpview(simeventsbhelp);
  wires:
  NumA/1 -> Divide/1
  Divide/1 -> ThroughPutA/1
  Digital Clock/1 -> Divide/2

== system sedemo_batch_production/Data Analysis/Compute Throughput B/AAA___ ==

== system sedemo_batch_production/Data Analysis/Compute Throughput B/__fcn_ss__ ==
  NumB : Inport  LoadFcn=des_subsysteminport(gcb, 'load');  InitFcn=des_subsysteminport(gcb, 'init');  StartFcn=des_subsysteminport(gcb, 'start');  StopFcn=des_subsysteminport(gcb, 'stop');  OutDataType=sfix(16)  OutScaling=2^0  mask(Discrete Event Inport){PermitSubsystemEvents=on, TypeOfEvent=Sample time hit, SignalEdgeOption=Rising, SpecifyEventPriority=off, PrioritySubsystemEvent=20}
      mask prompts: PermitSubsystemEvents "Execute subsystem upon signal-based events"; TypeOfEvent "Type of signal-based event:"; SignalEdgeOption "Type of change in signal value:"; SpecifyEventPriority "Resolve simultaneous signal updates according to event priority"; PrioritySubsystemEvent "Event priority:"
      mask help: Input port for a Discrete Event Subsystem block. This block can conditionally execute the subsystem upon signal-based events that meet specified criteria.
      mask init:
      | des_subsystemmask(gcb, 'init','apply')
      settings: CopyFcn=des_subsysteminport(gcb, 'copy');  DeleteFcn=des_subsysteminport(gcb, 'delete');  UndoDeleteFcn=des_subsysteminport(gcb, 'undodelete');  ModelCloseFcn=des_subsysteminport(gcb, 'modelclose');  PreSaveFcn=des_subsysteminport(gcb, 'presave');  NameChangeFcn=des_subsysteminport(gcb, 'namechange');  ParentCloseFcn=des_subsysteminport(gcb, 'parentclose');
      mask Help: helpview(simeventsbhelp);
      mask StyleString: checkbox,popup(Change in signal|Trigger|Sample time hit),popup(Rising|Falling|Either),checkbox,edit
      mask CallbackString: des_subsystemmask(gcb, 'cbPermitSubsystemEvents', 'noapply');|des_subsystemmask(gcb,'cbTypeOfEvent','noapply');||des_subsystemmask(gcb, 'cbSpecifyEventPriority', 'noapply');|
  Subsystem Configuration : TriggerPort  TriggerType=function-call
      settings: CopyFcn=des_subsystemconfigblock(gcb, 'copy');  DeleteFcn=des_subsystemconfigblock(gcb, 'delete');  UndoDeleteFcn=des_subsystemconfigblock(gcb, 'undodelete');
      mask Type: Subsystem Configuration
      mask Description: Configuration for a Discrete Event Subsystem block. Every discrete event subsystem window must contain exactly one copy of this configuration block. Do not delete this block.
      mask Help: helpview(simeventsbhelp);
      mask Display: disp('Do Not Delete');
  Digital Clock : DigitalClock  SampleTime=-1
  Divide : Product  Inputs=*/  OutDataType=sfix(16)  OutScaling=2^-10
  ThroughPutB : Outport  LoadFcn=des_subsystemoutport(gcb, 'load');  InitFcn=des_subsystemoutport(gcb, 'init');  StartFcn=des_subsystemoutport(gcb, 'start');  StopFcn=des_subsystemoutport(gcb, 'stop');  OutDataType=sfix(16)  OutScaling=2^0
      settings: CopyFcn=des_subsystemoutport(gcb, 'copy');  DeleteFcn=des_subsystemoutport(gcb, 'delete');  UndoDeleteFcn=des_subsystemoutport(gcb, 'undodelete');  ModelCloseFcn=des_subsystemoutport(gcb, 'modelclose');  PreSaveFcn=des_subsystemoutport(gcb, 'presave');  NameChangeFcn=des_subsystemoutport(gcb, 'namechange');  ParentCloseFcn=des_subsystemoutport(gcb, 'parentclose');
      mask Type: Discrete Event Outport
      mask Description: Provide an output port for a Discrete Event Subsystem block.
      mask Help: helpview(simeventsbhelp);
  wires:
  Digital Clock/1 -> Divide/2
  Divide/1 -> ThroughPutB/1
  NumB/1 -> Divide/1

== system sedemo_batch_production/Batch Reactors/Compute Utilization/Discrete Event Subsystem/AAA___ ==

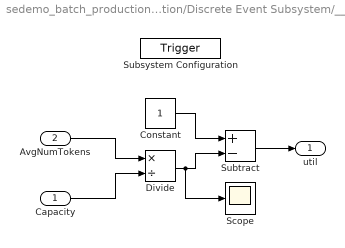
== system sedemo_batch_production/Batch Reactors/Compute Utilization/Discrete Event Subsystem/__fcn_ss__ ==
  Capacity : Inport  LoadFcn=des_subsysteminport(gcb, 'load');  InitFcn=des_subsysteminport(gcb, 'init');  StartFcn=des_subsysteminport(gcb, 'start');  StopFcn=des_subsysteminport(gcb, 'stop');  OutDataType=sfix(16)  OutScaling=2^0  mask(Discrete Event Inport){PermitSubsystemEvents=off, TypeOfEvent=Sample time hit, SignalEdgeOption=Rising, SpecifyEventPriority=off, PrioritySubsystemEvent=20}
      mask prompts: PermitSubsystemEvents "Execute subsystem upon signal-based events"; TypeOfEvent "Type of signal-based event:"; SignalEdgeOption "Type of change in signal value:"; SpecifyEventPriority "Resolve simultaneous signal updates according to event priority"; PrioritySubsystemEvent "Event priority:"
      mask help: Input port for a Discrete Event Subsystem block. This block can conditionally execute the subsystem upon signal-based events that meet specified criteria.
      mask init:
      | des_subsystemmask(gcb, 'init','apply')
      settings: CopyFcn=des_subsysteminport(gcb, 'copy');  DeleteFcn=des_subsysteminport(gcb, 'delete');  UndoDeleteFcn=des_subsysteminport(gcb, 'undodelete');  ModelCloseFcn=des_subsysteminport(gcb, 'modelclose');  PreSaveFcn=des_subsysteminport(gcb, 'presave');  NameChangeFcn=des_subsysteminport(gcb, 'namechange');  ParentCloseFcn=des_subsysteminport(gcb, 'parentclose');
      mask Help: helpview(simeventsbhelp);
      mask StyleString: checkbox,popup(Change in signal|Trigger|Sample time hit),popup(Rising|Falling|Either),checkbox,edit
      mask CallbackString: des_subsystemmask(gcb, 'cbPermitSubsystemEvents', 'noapply');|des_subsystemmask(gcb,'cbTypeOfEvent','noapply');||des_subsystemmask(gcb, 'cbSpecifyEventPriority', 'noapply');|
  AvgNumTokens : Inport  LoadFcn=des_subsysteminport(gcb, 'load');  InitFcn=des_subsysteminport(gcb, 'init');  StartFcn=des_subsysteminport(gcb, 'start');  StopFcn=des_subsysteminport(gcb, 'stop');  Port=2  OutDataType=sfix(16)  OutScaling=2^0  mask(Discrete Event Inport){PermitSubsystemEvents=on, TypeOfEvent=Sample time hit, SignalEdgeOption=Rising, SpecifyEventPriority=off, PrioritySubsystemEvent=20}
      mask prompts: PermitSubsystemEvents "Execute subsystem upon signal-based events"; TypeOfEvent "Type of signal-based event:"; SignalEdgeOption "Type of change in signal value:"; SpecifyEventPriority "Resolve simultaneous signal updates according to event priority"; PrioritySubsystemEvent "Event priority:"
      mask help: Input port for a Discrete Event Subsystem block. This block can conditionally execute the subsystem upon signal-based events that meet specified criteria.
      mask init:
      | des_subsystemmask(gcb, 'init','apply')
      settings: CopyFcn=des_subsysteminport(gcb, 'copy');  DeleteFcn=des_subsysteminport(gcb, 'delete');  UndoDeleteFcn=des_subsysteminport(gcb, 'undodelete');  ModelCloseFcn=des_subsysteminport(gcb, 'modelclose');  PreSaveFcn=des_subsysteminport(gcb, 'presave');  NameChangeFcn=des_subsysteminport(gcb, 'namechange');  ParentCloseFcn=des_subsysteminport(gcb, 'parentclose');
      mask Help: helpview(simeventsbhelp);
      mask StyleString: checkbox,popup(Change in signal|Trigger|Sample time hit),popup(Rising|Falling|Either),checkbox,edit
      mask CallbackString: des_subsystemmask(gcb, 'cbPermitSubsystemEvents', 'noapply');|des_subsystemmask(gcb,'cbTypeOfEvent','noapply');||des_subsystemmask(gcb, 'cbSpecifyEventPriority', 'noapply');|
  Subsystem Configuration : TriggerPort  TriggerType=function-call
      settings: CopyFcn=des_subsystemconfigblock(gcb, 'copy');  DeleteFcn=des_subsystemconfigblock(gcb, 'delete');  UndoDeleteFcn=des_subsystemconfigblock(gcb, 'undodelete');
      mask Type: Subsystem Configuration
      mask Description: Configuration for a Discrete Event Subsystem block. Every discrete event subsystem window must contain exactly one copy of this configuration block. Do not delete this block.
      mask Help: helpview(simeventsbhelp);
      mask Display: disp('Do Not Delete');
  Constant : Constant  OutDataType=sfix(16)  OutScaling=2^0
  Divide : Product  Inputs=*/  OutDataType=sfix(16)  OutScaling=2^-10
  Scope : Scope
  Subtract : Sum  Inputs=+-  OutDataType=sfix(16)  OutScaling=2^-10
  util : Outport  LoadFcn=des_subsystemoutport(gcb, 'load');  InitFcn=des_subsystemoutport(gcb, 'init');  StartFcn=des_subsystemoutport(gcb, 'start');  StopFcn=des_subsystemoutport(gcb, 'stop');  OutDataType=sfix(16)  OutScaling=2^0
      settings: CopyFcn=des_subsystemoutport(gcb, 'copy');  DeleteFcn=des_subsystemoutport(gcb, 'delete');  UndoDeleteFcn=des_subsystemoutport(gcb, 'undodelete');  ModelCloseFcn=des_subsystemoutport(gcb, 'modelclose');  PreSaveFcn=des_subsystemoutport(gcb, 'presave');  NameChangeFcn=des_subsystemoutport(gcb, 'namechange');  ParentCloseFcn=des_subsystemoutport(gcb, 'parentclose');
      mask Type: Discrete Event Outport
      mask Description: Provide an output port for a Discrete Event Subsystem block.
      mask Help: helpview(simeventsbhelp);
  wires:
  Capacity/1 -> Divide/2
  AvgNumTokens/1 -> Divide/1
  Constant/1 -> Subtract/1
  Divide/1 -> Subtract/2, Scope/1
  Subtract/1 -> util/1
